simulink model "sbd_r2015b"  (R2016b)
settings: Solver=FixedStepDiscrete  StartTime=0.0  StopTime=99999  RelTol=1e-3  EnableMultiTasking=on
undefined symbols (not defined in the file): gray, Rec, SDTV
libraries: visionstatistics x2, simulink x2, visiontextngfix x2, visionconversions x2, dspvision x1, dspsnks4 x1
settings Model: Creator=leszczuk  LastModifiedBy=miklesz
settings DataIOCC: LimitDataPoints=on  SaveFormat=Array  SignalLoggingSaveFormat=ModelDataLogs
settings OptimizationCC: ExpressionDepthLimit=2147483647  InitFltsAndDblsToZero=on  LifeSpan=inf
settings DebuggingCC: SaveWithParameterizedLinksMsg=none  UnderspecifiedInitializationDetection=Classic  MergeDetectMultiDrivingBlocksExec=none  ParameterPrecisionLossMsg=none  FcnCallInpInsideContextMsg=warning  AllowSymbolicDim=off  StateNameClashWarn=warning  SFUnexpectedBacktrackingDiag=warning  SFNoUnconditionalDefaultTransitionDiag=warning  SFExecutionAtInitializationDiag=none
settings HardwareCC: ProdBitPerPointer=32  ProdBitPerSizeT=32  ProdBitPerPtrDiffT=32  ProdLargestAtomicFloat=None  ProdIntDivRoundTo=Undefined  ProdEndianess=Unspecified  ProdWordSize=32  ProdHWDeviceType=32-bit Generic
settings ModelReferenceCC: PropagateSignalLabelsOutOfModel=off
settings GRTTargetCC: TargetFcnLib=ansi_tfl_tmw.mat  TargetLangStandard=C89/C90 (ANSI)  GeneratePreprocessorConditionals=Disable all  CombineOutputUpdateFcns=off  GRTInterface=on
settings ConfigComp: CovMetricSettings=dw  CovHtmlReporting=on  CovSaveCumulativeToWorkspaceVar=on  CovSaveSingleToWorkspaceVar=on  CovExternalEMLEnable=off

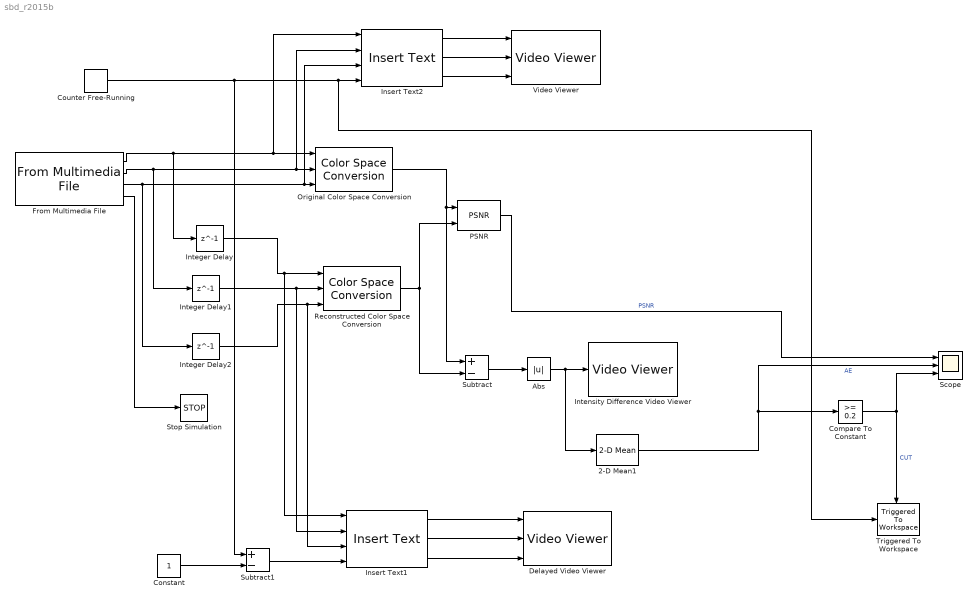
== system sbd_r2015b ==
  2-D Mean1 : visionstatistics/2-D Mean  run=off  reset_popup=None  directionMode=Entire input  dimension=1  treatSBRowAsCol=on  roiEnable=off  roiType=Rectangles  roiPortion=Entire ROI  roiOutput=Individual statistics for each ROI  roiFlag=off  outputDataTypeStr=Inherit: Same as accumulator  outputLastDataTypeStr=Inherit: Same as accumulator  outputMin=[]  outputMax=[]  accumMode=Binary point scaling  accumWordLength=32  accumFracLength=0  accumDataTypeStr=fixdt([],32,0)  accumLastDataTypeStr=fixdt([],32,0)  roundingMode=Floor  overflowMode=off
  Abs : Abs
  Compare To Constant : simulink/Logic and Bit Operations/Compare To Constant  relop=>=  const=0.2  OutDataTypeStr=uint8  ZeroCross=off
  Constant : Constant
  Counter Free-Running : simulink/Sources/Counter Free-Running  NumBits=16  tsamp=-1
  Delayed Video Viewer : VideoViewer  imagePorts=separate color signals  colormapValue=gray(256)  FigPos=[43 508 454 294]  AxisZoom=off  trueSizedOnce=on
  From Multimedia File : dspvision/From Multimedia File  inputFilename=/Users/miklesz/OneDrive/Teaching/AMIPaC/10 (19) Shot Boundary Detection (SBD)/50028.mpg  loop=on  numPlays=1  outputStreams=Video only  videoDataType=single  audioDataType=int16  inheritSampleTime=on  userDefinedSampleTime=1/30  noAudioOutput=off  isIntensityVideo=off  fourcc=RGB  colorVideoFormat=Separate color signals  outputEOF=on  dataOrg=Column-major  audioFrameSize=1024  computeAudioFrameSize=off  outSamplingMode=Frame based
  Insert Text1 : visiontextngfix/Insert Text  inputType=Obsolete  theText='postFNum=%d'  getTextLocFrom=Specify via dialog  textLoc=[1 1]  getTextColorFrom=Specify via dialog  textColor=[255 255 0]  getTextIntensityFrom=Specify via dialog  textIntensity=0  getTextOpacityFrom=Specify via dialog  textOpacity=1.0  dummyVar2=0  dummyVar3=0  dummyVar4=0  imagePorts=Separate color signals  isInputTransposed=off  fontFace=LucidaSansRegular  dummyVar1=0  blockFontSize=12  antiAliased=on
  Insert Text2 : visiontextngfix/Insert Text  inputType=Obsolete  theText='preFNum=%d'  getTextLocFrom=Specify via dialog  textLoc=[1 1]  getTextColorFrom=Specify via dialog  textColor=[255 255 0]  getTextIntensityFrom=Specify via dialog  textIntensity=0  getTextOpacityFrom=Specify via dialog  textOpacity=1.0  dummyVar2=0  dummyVar3=0  dummyVar4=0  imagePorts=Separate color signals  isInputTransposed=off  fontFace=LucidaSansRegular  dummyVar1=0  blockFontSize=12  antiAliased=on
  Integer Delay : Delay  DelayLength=1  InputProcessing=Inherited
  Integer Delay1 : Delay  DelayLength=1  InputProcessing=Inherited
  Integer Delay2 : Delay  DelayLength=1  InputProcessing=Inherited
  Intensity Difference Video Viewer : VideoViewer  colormapValue=gray(256)  FigPos=[395 831 454 294]  AxisZoom=off  trueSizedOnce=on
  Original Color Space Conversion : visionconversions/Color Space  Conversion  conversion=Obsolete  conversionActive=R'G'B' to intensity  wp_str=D65  rec=Rec. 601 (SDTV)  sys=1125/60/2:1  imagePorts=Separate color signals
  PSNR : visionstatistics/PSNR
  Reconstructed Color Space Conversion : visionconversions/Color Space  Conversion  conversion=Obsolete  conversionActive=R'G'B' to intensity  wp_str=D65  rec=Rec. 601 (SDTV)  sys=1125/60/2:1  imagePorts=Separate color signals
  Scope : Scope  NumInputPorts=3
  Stop Simulation : Stop
  Subtract : Sum  Inputs=+-
  Subtract1 : Sum  Inputs=+-  OutDataTypeStr=int16
  Triggered To Workspace : dspsnks4/Triggered To Workspace  TriggerType=Rising edge  VariableName=autoPostFNum  Buffer=1000
      settings: FixptAsFi=off
  Video Viewer : VideoViewer  imagePorts=separate color signals  colormapValue=gray(256)  FigPos=[767 502 454 294]  AxisZoom=off  trueSizedOnce=on
  wires:
  PSNR/1 -> Scope/1  "PSNR"
  From Multimedia File/1 -> Integer Delay/1, Insert Text2/1, Original Color Space Conversion/1
  Original Color Space Conversion/1 -> Subtract/1, PSNR/1
  Reconstructed Color Space Conversion/1 -> PSNR/2, Subtract/2
  From Multimedia File/2 -> Integer Delay1/1, Insert Text2/2, Original Color Space Conversion/2
  From Multimedia File/3 -> Integer Delay2/1, Insert Text2/3, Original Color Space Conversion/3
  Integer Delay1/1 -> Insert Text1/2, Reconstructed Color Space Conversion/2
  2-D Mean1/1 -> Scope/2, Compare To Constant/1  "AE"
  Subtract/1 -> Abs/1
  Abs/1 -> 2-D Mean1/1, Intensity Difference Video Viewer/1
  Integer Delay2/1 -> Insert Text1/3, Reconstructed Color Space Conversion/3
  Integer Delay/1 -> Insert Text1/1, Reconstructed Color Space Conversion/1
  Insert Text1/1 -> Delayed Video Viewer/1
  Insert Text1/2 -> Delayed Video Viewer/2
  Insert Text1/3 -> Delayed Video Viewer/3
  Insert Text2/1 -> Video Viewer/1
  Insert Text2/2 -> Video Viewer/2
  Insert Text2/3 -> Video Viewer/3
  Counter Free-Running/1 -> Subtract1/1, Insert Text2/4, Triggered To Workspace/1
  Subtract1/1 -> Insert Text1/4
  Constant/1 -> Subtract1/2
  Compare To Constant/1 -> Scope/3, Triggered To Workspace/Trigger  "CUT"
  From Multimedia File/4 -> Stop Simulation/1
